simulink model "Control - Scenario 6"  (R2019b)
settings: Solver=VariableStepAuto  StartTime=0.0  StopTime=10.0  RelTol=1e-3
undefined symbols (not defined in the file): DENd, DENd_pf, NUMd, NUMd_pf, T_6
libraries: cstblocks x26
settings Model: Creator=Gioele  LastModifiedBy=Gioele

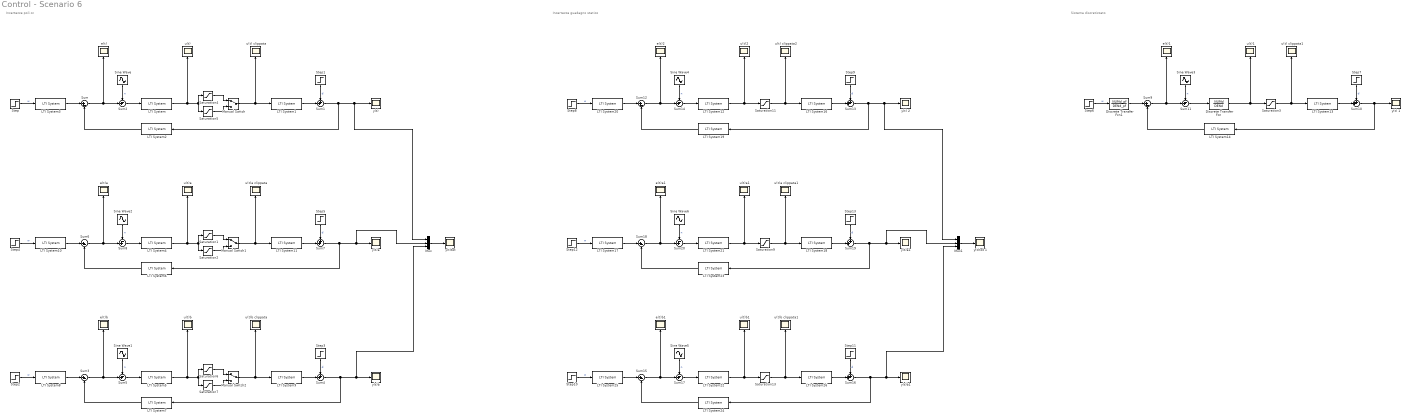
== system Control - Scenario 6 ==
  note: Incertezze guadagno statico
  note: Sistema discretizzato
  note: Incertezze poli cc
  Discrete Transfer Fcn : DiscreteTransferFcn  Numerator=NUMd  Denominator=DENd  SampleTime=T_6
  Discrete Transfer Fcn1 : DiscreteTransferFcn  Numerator=NUMd_pf  Denominator=DENd_pf  SampleTime=T_6
  LTI System{,4..5,12,21..22} (6 alike) : cstblocks/LTI System  sys=R_6  IC=[]
  LTI System1 : cstblocks/LTI System  sys=G  IC=[]
  LTI System{3,8,10,17,20,25} (6 alike) : cstblocks/LTI System  sys=Rpf_6  IC=[]
  LTI System11 : cstblocks/LTI System  sys=Ga  IC=[]
  LTI System13 : cstblocks/LTI System  sys=G  IC=[]
  LTI System{2,6..7,14,19,23..24} (7 alike) : cstblocks/LTI System  sys=Haa_6  IC=[]
  LTI System16 : cstblocks/LTI System  sys=G  IC=[]
  LTI System18 : cstblocks/LTI System  sys=Gf  IC=[]
  LTI System26 : cstblocks/LTI System  sys=Gg  IC=[]
  LTI System9 : cstblocks/LTI System  sys=Gb  IC=[]
  Manual Switch : ManualSwitch
  Manual Switch1 : ManualSwitch
  Manual Switch2 : ManualSwitch
  Mux : Mux  Inputs=3
  Mux1 : Mux  Inputs=3
  Saturation1 : Saturate  UpperLimit=5.67  LowerLimit=-5.67
  Saturation{2..3,5,7,9,11,13} (7 alike) : Saturate  UpperLimit=8  LowerLimit=-8
  Saturation4 : Saturate  UpperLimit=5.67  LowerLimit=-5.67
  Saturation6 : Saturate  UpperLimit=5.67  LowerLimit=-5.67
  Sine Wave{,1..6} (7 alike) : Sin  Amplitude=0.005  Frequency=2000  SampleTime=0
  Step{,2,4,6,8,10,12} (7 alike) : Step  Time=0  After=2  SampleTime=0
  Step{1,3,5,7,9,11,13} (7 alike) : Step  Time=0  After=0.1  SampleTime=0
  Sum{,3,6,9,12,15,18} (7 alike) : Sum  Inputs=|+-
  Sum{1,4,7,10,13,16,19} (7 alike) : Sum  Inputs=++|
  Sum{2,5,8,11,14,17,20} (7 alike) : Sum  Inputs=-+|
  e(t) : Scope
  e(t)1 : Scope
  e(t)2 : Scope
  e(t)a : Scope
  e(t)a1 : Scope
  e(t)b : Scope
  e(t)b1 : Scope
  u(t) : Scope
  u(t) clippata : Scope
  u(t) clippata1 : Scope
  u(t) clippata2 : Scope
  u(t)1 : Scope
  u(t)2 : Scope
  u(t)a : Scope
  u(t)a clippata : Scope
  u(t)a clippata1 : Scope
  u(t)a1 : Scope
  u(t)b : Scope
  u(t)b clippata : Scope
  u(t)b clippata1 : Scope
  u(t)b1 : Scope
  "y(t) " : Scope
  y(t) 1 : Scope
  y(t) 2 : Scope
  y(t)a : Scope
  y(t)a1 : Scope
  y(t)b : Scope
  y(t)b1 : Scope
  "y(t)tot " : Scope
  y(t)tot 1 : Scope
  wires:
  Manual Switch1/1 -> LTI System11/1, u(t)a clippata/1
  LTI System6/1 -> Sum6/2
  LTI System3/1 -> Sum/1
  Step4/1 -> LTI System10/1  "w"
  Sum6/1 -> Sum8/2, e(t)a/1
  Sum4/1 -> LTI System7/1, y(t)b/1, Mux/3
  Sum8/1 -> LTI System4/1
  Sum5/1 -> LTI System5/1
  LTI System7/1 -> Sum3/2
  LTI System11/1 -> Sum7/2
  LTI System9/1 -> Sum4/2
  LTI System2/1 -> Sum/2
  Step5/1 -> Sum7/1  "d"
  Sum7/1 -> y(t)a/1, Mux/2, LTI System6/1
  Sine Wave2/1 -> Sum8/1  "n"
  Sine Wave1/1 -> Sum5/1  "n"
  Sum2/1 -> LTI System/1
  Manual Switch/1 -> LTI System1/1, u(t) clippata/1
  Sum1/1 -> "y(t) "/1, Mux/1, LTI System2/1
  LTI System1/1 -> Sum1/2
  LTI System10/1 -> Sum6/1
  Step2/1 -> LTI System8/1  "w"
  Mux/1 -> "y(t)tot "/1
  LTI System8/1 -> Sum3/1
  Sum3/1 -> e(t)b/1, Sum5/2
  Sine Wave/1 -> Sum2/1  "n"
  Sum/1 -> e(t)/1, Sum2/2
  Step/1 -> LTI System3/1  "w"
  Manual Switch2/1 -> LTI System9/1, u(t)b clippata/1
  Step3/1 -> Sum4/1  "d"
  Step1/1 -> Sum1/1  "d"
  Step7/1 -> Sum10/1  "d"
  LTI System14/1 -> Sum9/2
  Discrete Transfer Fcn/1 -> u(t)1/1, Saturation3/1
  Saturation3/1 -> LTI System13/1, u(t) clippata1/1
  Step6/1 -> Discrete Transfer Fcn1/1  "w"
  Sum9/1 -> e(t)1/1, Sum11/2
  Sine Wave3/1 -> Sum11/1  "n"
  Sum10/1 -> y(t) 1/1, LTI System14/1
  Sum11/1 -> Discrete Transfer Fcn/1
  LTI System13/1 -> Sum10/2
  LTI System/1 -> Saturation5/1, Saturation4/1, u(t)/1
  Saturation4/1 -> Manual Switch/1
  Saturation5/1 -> Manual Switch/2
  LTI System4/1 -> Saturation2/1, Saturation1/1, u(t)a/1
  Saturation1/1 -> Manual Switch1/1
  Saturation2/1 -> Manual Switch1/2
  LTI System5/1 -> Saturation7/1, Saturation6/1, u(t)b/1
  Saturation6/1 -> Manual Switch2/1
  Saturation7/1 -> Manual Switch2/2
  Sum17/1 -> LTI System22/1
  Sum18/1 -> Sum20/2, e(t)a1/1
  Saturation9/1 -> LTI System18/1, u(t)a clippata1/1
  Step12/1 -> LTI System17/1  "w"
  Sum16/1 -> LTI System24/1, y(t)b1/1, Mux1/3
  LTI System22/1 -> u(t)b1/1, Saturation13/1
  Sine Wave5/1 -> Sum17/1  "n"
  Sum12/1 -> e(t)2/1, Sum14/2
  LTI System12/1 -> Saturation11/1, u(t)2/1
  LTI System21/1 -> Saturation9/1, u(t)a1/1
  Sum15/1 -> e(t)b1/1, Sum17/2
  Saturation13/1 -> LTI System26/1, u(t)b clippata1/1
  Sine Wave4/1 -> Sum14/1  "n"
  LTI System23/1 -> Sum18/2
  Step11/1 -> Sum16/1  "d"
  Step9/1 -> Sum13/1  "d"
  Sum19/1 -> y(t)a1/1, Mux1/2, LTI System23/1
  Sum14/1 -> LTI System12/1
  LTI System26/1 -> Sum16/2
  Step13/1 -> Sum19/1  "d"
  LTI System24/1 -> Sum15/2
  LTI System16/1 -> Sum13/2
  Saturation11/1 -> LTI System16/1, u(t) clippata2/1
  Sum20/1 -> LTI System21/1
  Step10/1 -> LTI System25/1  "w"
  Step8/1 -> LTI System20/1  "w"
  Sine Wave6/1 -> Sum20/1  "n"
  Sum13/1 -> y(t) 2/1, Mux1/1, LTI System19/1
  LTI System19/1 -> Sum12/2
  LTI System17/1 -> Sum18/1
  LTI System20/1 -> Sum12/1
  LTI System18/1 -> Sum19/2
  LTI System25/1 -> Sum15/1
  Mux1/1 -> y(t)tot 1/1
  Discrete Transfer Fcn1/1 -> Sum9/1
